simulink model "final_test"  (R2022b)
settings: Solver=VariableStepAuto  StartTime=0.0  StopTime=50  RelTol=1e-3
settings Model: Creator=anver  LastModifiedBy=anver

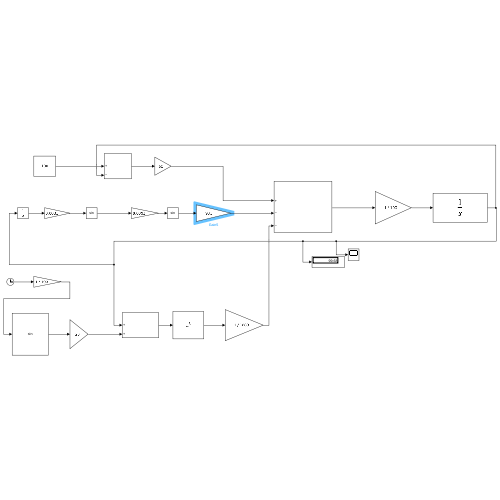
[thumbnail: Simulink's stored preview of the top-level diagram]
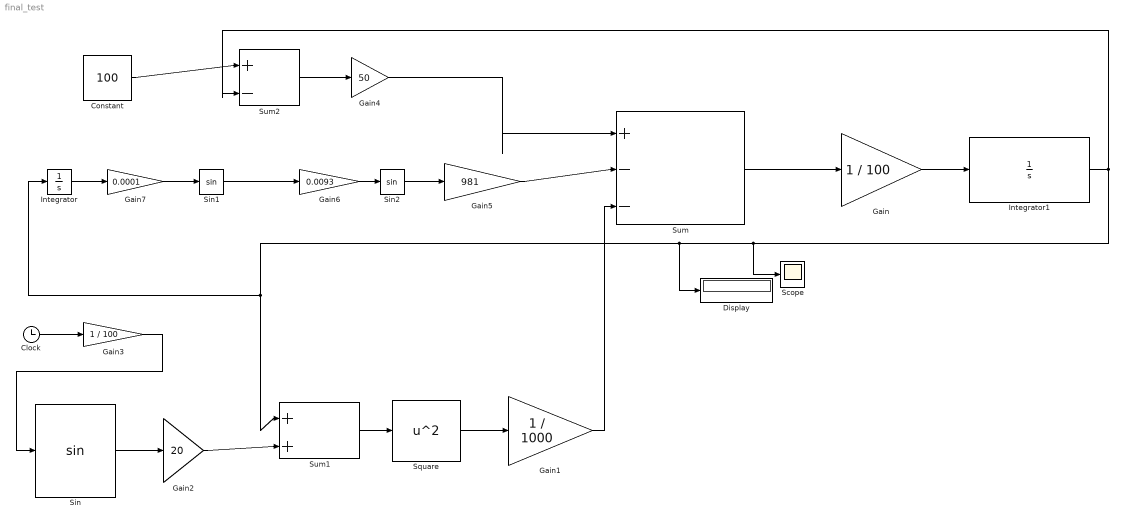
== system final_test ==
  Clock : Clock
  Constant : Constant  Value=100
  Display : Display
  Gain : Gain  Gain=1 / 100
  Gain1 : Gain  Gain=1 / 1000
  Gain2 : Gain  Gain=20
  Gain3 : Gain  Gain=1 / 100
  Gain4 : Gain  Gain=50
  Gain5 : Gain  Gain=981
  Gain6 : Gain  Gain=0.0093
  Gain7 : Gain  Gain=0.0001
  Integrator : Integrator
  Integrator1 : Integrator
  Scope : Scope
  Sin : Trigonometry
  Sin1 : Trigonometry
  Sin2 : Trigonometry
  Square : Math  Operator=square
  Sum : Sum  Inputs=|+--
  Sum1 : Sum  Inputs=|++
  Sum2 : Sum  Inputs=|+-
  wires:
  Gain/1 -> Integrator1/1
  Sum/1 -> Gain/1
  Gain1/1 -> Sum/3
  Square/1 -> Gain1/1
  Sum1/1 -> Square/1
  Gain2/1 -> Sum1/2
  Sin/1 -> Gain2/1
  Integrator1/1 -> Sum2/2, Scope/1, Display/1, Integrator/1, Sum1/1
  Clock/1 -> Gain3/1
  Gain3/1 -> Sin/1
  Sum2/1 -> Gain4/1
  Gain4/1 -> Sum/1
  Constant/1 -> Sum2/1
  Gain5/1 -> Sum/2
  Sin1/1 -> Gain6/1
  Gain7/1 -> Sin1/1
  Integrator/1 -> Gain7/1
  Gain6/1 -> Sin2/1
  Sin2/1 -> Gain5/1
